simulink model "TestHiTechnicSensors"  (Simulink 6.4)
settings: Solver=FixedStepDiscrete  SolverMode=SingleTasking  StartTime=0  StopTime=inf  FixedStep=0.001  RelTol=1e-3
libraries: ecrobot_nxt_lib x8
settings Model: Creator=tchikama  LastModifiedBy=tchikama  ProdHWDeviceType=ARM7
settings DataIOCC: SaveOutput=off  SignalLogging=off  SaveTime=off
settings OptimizationCC: InlineParams=on  InlineInvariantSignals=on  RollThreshold=2  StateBitsets=on  DataBitsets=on  UseTempVars=on  InitFltsAndDblsToZero=off  NoFixptDivByZeroProtection=on  EfficientFloat2IntCast=on  OptimizeModelRefInitCode=on  LifeSpan=1
settings DebuggingCC: ConsistencyChecking=warning  SignalInfNanChecking=warning  ReadBeforeWriteMsg=DisableAll  WriteAfterWriteMsg=DisableAll  WriteAfterReadMsg=DisableAll  AlgebraicLoopMsg=error  CheckExecutionContextPreStartOutputMsg=on  CheckExecutionContextRuntimeOutputMsg=on  SolverPrmCheckMsg=none  SingleTaskRateTransMsg=warning  TasksWithSamePriorityMsg=none  IntegerOverflowMsg=error  ParameterPrecisionLossMsg=none  UnconnectedInputMsg=error  UnconnectedOutputMsg=error  UnconnectedLineMsg=error  UniqueDataStoreMsg=error  BusObjectLabelMismatch=error  RootOutportRequireBusObject=error  ModelReferenceIOMsg=warning  ModelReferenceVersionMismatchMessage=warning  ModelReferenceIOMismatchMessage=warning
settings HardwareCC: ProdIntDivRoundTo=Zero  ProdEndianess=LittleEndian  ProdHWDeviceType=ARM7  TargetHWDeviceType=32-bit Generic
settings ModelReferenceCC: ModelReferenceNumInstancesAllowed=Single
settings RTWCC: SystemTargetFile=ert.tlc  GenCodeOnly=on  GenerateMakefile=off  TemplateMakefile=ert_default_tmf  Description=Real-Time Workshop Embedded Coder (no auto configuration)  GenerateReport=on  RTWVerbose=off  ProcessScript=ert_make_rtw_hook  IncludeHyperlinkInReport=on  LaunchReport=on
settings CodeAppCC: ForceParamTrailComments=on  IgnoreCustomStorageClasses=off  SFDataObjDesc=on  PrefixModelToSubsysFcnNames=off  CustomSymbolStrGlobalVar=rt$N$M  CustomSymbolStrType=$N$M  CustomSymbolStrFcn=$N$M$F  CustomSymbolStrMacro=$N$M  InsertBlockDesc=on
settings ERTTargetCC: TargetFcnLib=ansi_tfl_tmw.mat  GenFloatMathFcnCalls=GNU  IncludeMdlTerminateFcn=off  SuppressErrorStatus=on  IncludeERTFirstTime=on  SupportAbsoluteTime=off  SupportNonFinite=off  SupportComplex=off  PurelyIntegerCode=on  InlinedParameterPlacement=NonHierarchical  RootIOFormat=Structure reference  ERTCustomFileTemplate=example_file_process.tlc  InitialValueSource=Model

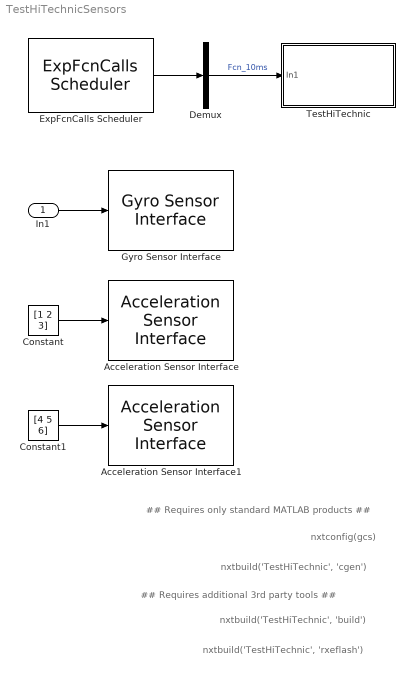
== system TestHiTechnicSensors ==
  note: nxtbuild('TestHiTechnic', 'build')
  note: nxtbuild('TestHiTechnic', 'rxeflash')
  note: nxtbuild('TestHiTechnic', 'cgen')
  note: ## Requires only standard MATLAB products ##
  note: ## Requires additional 3rd party tools ##
  note: nxtconfig(gcs)
  In1 : Inport
  Acceleration Sensor Interface : ecrobot_nxt_lib/Acceleration Sensor Interface  SystemSampleTime=-1  ip=S3
  Acceleration Sensor Interface1 : ecrobot_nxt_lib/Acceleration Sensor Interface  SystemSampleTime=-1  ip=S4
  Constant : Constant  Value=[1 2 3]  OutDataType=sfix(16)  ConRadixGroup=Use specified scaling  OutScaling=2^0  SampleTime=inf  FramePeriod=inf
  Constant1 : Constant  Value=[4 5 6]  OutDataType=sfix(16)  ConRadixGroup=Use specified scaling  OutScaling=2^0  SampleTime=inf  FramePeriod=inf
  Demux : Demux  Outputs=1
  ExpFcnCalls Scheduler : ecrobot_nxt_lib/ExpFcnCalls Scheduler  fcname='Fcn_10ms'  fctrigger=[10]  ts=0.001  platform=OSEK  stacksize=[512]  bd_mode=Slave
  Gyro Sensor Interface : ecrobot_nxt_lib/Gyro Sensor Interface  SystemSampleTime=-1  ip=S1
  TestHiTechnic : Subsystem
  wires:
  ExpFcnCalls Scheduler/1 -> Demux/1
  Demux/1 -> TestHiTechnic/1(In1)  "Fcn_10ms"
  In1/1 -> Gyro Sensor Interface/1
  Constant/1 -> Acceleration Sensor Interface/1
  Constant1/1 -> Acceleration Sensor Interface1/1

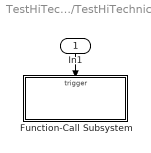
== system TestHiTechnicSensors/TestHiTechnic ==
  In1 : Inport  Orientation=down
  Function-Call Subsystem : Subsystem  TreatAsAtomicUnit=on
  wires:
  In1/1 -> Function-Call Subsystem/Trigger

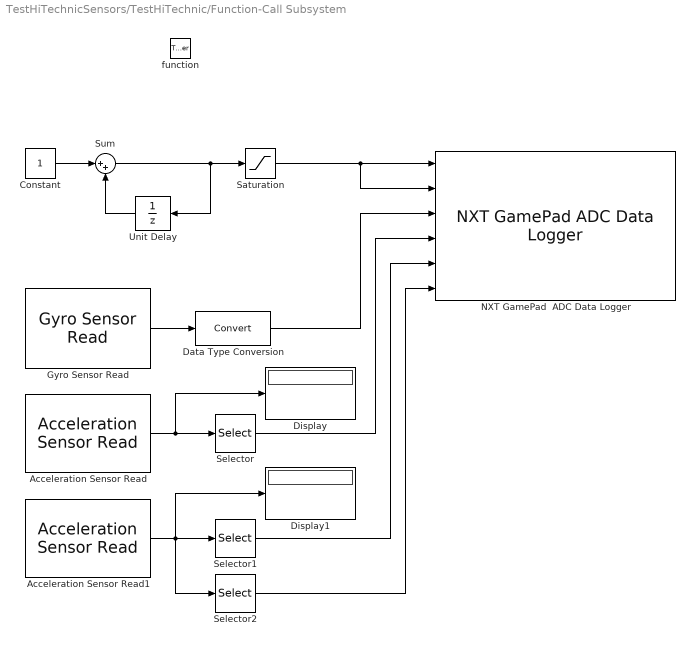
== system TestHiTechnicSensors/TestHiTechnic/Function-Call Subsystem ==
  function : TriggerPort  TriggerType=function-call
  Acceleration Sensor Read : ecrobot_nxt_lib/Acceleration Sensor Read  ip=S3
  Acceleration Sensor Read1 : ecrobot_nxt_lib/Acceleration Sensor Read  ip=S4
  Constant : Constant  Value=1  OutDataTypeMode=int8  OutDataType=sfix(16)  ConRadixGroup=Use specified scaling  OutScaling=2^0  SampleTime=inf  FramePeriod=inf
  Data Type Conversion : DataTypeConversion  OutDataTypeMode=int16
  Display : Display
  Display1 : Display
  Gyro Sensor Read : ecrobot_nxt_lib/Gyro Sensor Read  SystemSampleTime=-1  ip=S1
  NXT GamePad  ADC Data Logger : ecrobot_nxt_lib/NXT GamePad  ADC Data Logger
  Saturation : Saturate  UpperLimit=100  LowerLimit=-100
  Selector : Selector  IndexMode=Zero-based  Elements=0  InputPortWidth=3
  Selector1 : Selector  IndexMode=Zero-based  InputPortWidth=3
  Selector2 : Selector  IndexMode=Zero-based  Elements=2  InputPortWidth=3
  Sum : Sum  Inputs=|++
  Unit Delay : UnitDelay  Orientation=left  SampleTime=-1
  wires:
  Unit Delay/1 -> Sum/2
  Sum/1 -> Saturation/1, Unit Delay/1
  Constant/1 -> Sum/1
  Saturation/1 -> NXT GamePad  ADC Data Logger/1, NXT GamePad  ADC Data Logger/2
  Gyro Sensor Read/1 -> Data Type Conversion/1
  Selector/1 -> NXT GamePad  ADC Data Logger/4
  Selector1/1 -> NXT GamePad  ADC Data Logger/5
  Selector2/1 -> NXT GamePad  ADC Data Logger/6
  Data Type Conversion/1 -> NXT GamePad  ADC Data Logger/3
  Acceleration Sensor Read/1 -> Selector/1, Display/1
  Acceleration Sensor Read1/1 -> Selector1/1, Selector2/1, Display1/1
